simulink model "ClosedLoopPMSM_PID_asmo"  (R2023b)
settings: Solver=ode4  StartTime=0.0  StopTime=2.5  FixedStep=1e-6  RelTol=1e-4
InitFcn:
  | Vdc=24;
  | Rs=0.05734;
  | Ld=1.8166e-05;
  | Lq=1.8166e-05;
  | Ls=1.8166e-05;
  | pm=0.0185;
  | P=14;
  | B=1e-4;
  | J=2.94e-5;
  | Tpwm=30e-6;
  | 
  | fc=20;
  | mag_vel=100;
undefined symbols (not defined in the file): DiscIntNeverNeededParam
libraries: simulink x4, slpidlib x3, spsThreePhaseVIMeasurementLib x2, spsDCVoltageSourceLib x2, spsThreeLevelBridgeLib x1, spsUniversalBridgeLib x1, spsPermanentMagnetSynchronousMachineLib x1, sps_lib x1
settings Model: Creator=Admin  LastModifiedBy=Admin
settings SolverCC: AlgebraicLoopSolver=TrustRegion
settings DataIOCC: ReturnWorkspaceOutputs=off
settings OptimizationCC: LifeSpan=inf
settings DebuggingCC: UnconnectedInputMsg=warning  UnconnectedOutputMsg=warning  UnconnectedLineMsg=warning  SFUnexpectedBacktrackingDiag=warning  SFNoUnconditionalDefaultTransitionDiag=warning  ArithmeticOperatorsInVariantConditions=warning
settings ModelReferenceCC: EnableRefExpFcnMdlSchedulingChecks=on
settings SFSimCC: SimUseLocalCustomCode=off  CustomCodeUndefinedFunction=UseInterfaceOnly
settings RTWCC: RTWUseLocalCustomCode=off
settings CodeAppCC: StateflowObjectComments=on
settings GRTTargetCC: TargetLangStandard=C89/C90 (ANSI)
settings ConfigComp: CovMetricSettings=dw  CovSaveCumulativeToWorkspaceVar=on  CovSaveSingleToWorkspaceVar=on  CovExternalEMLEnable=off
settings SimscapeCC: SimscapeNormalizeSystem=off

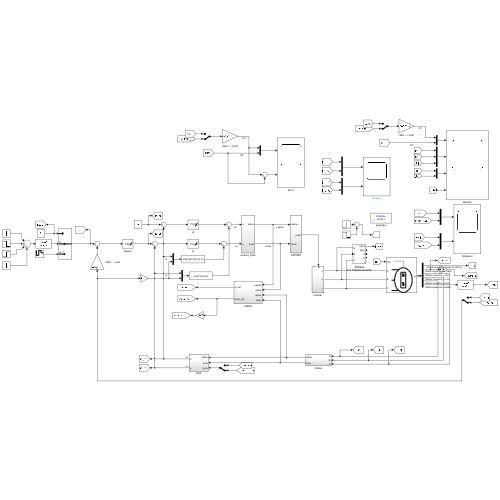
[thumbnail: Simulink's stored preview of the top-level diagram]
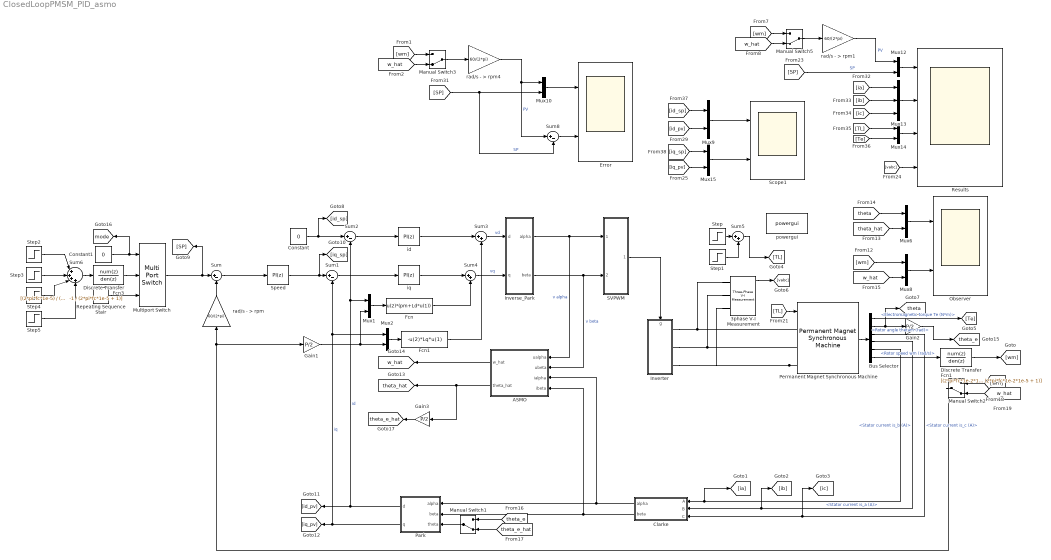
== system ClosedLoopPMSM_PID_asmo ==
  3phase V-I Measurement : spsThreePhaseVIMeasurementLib/Three-Phase V-I Measurement  VoltageMeasurement=phase-to-phase  SetLabelV=off  LabelV=Vabc  Vpu=off  VpuLL=off  CurrentMeasurement=yes  SetLabelI=off  LabelI=Iabc  Ipu=off  Pbase=100e6  Vbase=500e3  OutputType=Complex  PhasorSimulation=off  PSBequivalent=0
  ASMO : Subsystem
  Bus Selector : BusSelector  OutputSignals=Electromagnetic torque Te (N*m),Rotor angle thetam (rad),Stator current is_c (A),Stator current is_b (A),Stator current is_a (A),Rotor speed wm (rad/s)
  Clarke : Subsystem
  Constant : Constant  Value=0
  Constant1 : Constant  Value=0
  Discrete Transfer Fcn1 : DiscreteTransferFcn  Numerator=[(2*pi*fc*1e-2*1e-5) / (2*pi*fc*1e-2*1e-5 + 1)]  Denominator="[1   -1 / (2*pi*fc*1e-2*1e-5 + 1)]"
  Discrete Transfer Fcn3 : DiscreteTransferFcn  Numerator=[(2*pi*fc*1e-5) / (2*pi*fc*1e-5 + 1)]  Denominator="[1   -1 / (2*pi*fc*1e-5 + 1)]"
  Error : Scope  NumInputPorts=2
  Fcn : Fcn  Expr=u(2)*(pm+Ld*u(1))
  Fcn1 : Fcn  Expr=-u(2)*Lq*u(1)
  Gain1 : Gain  Gain=P/2
  Gain2 : Gain  Gain=P/2
  Gain3 : Gain  Gain=P/2
  Inverse_Park : Subsystem
  Inverter : Subsystem
      settings: PortSchema="{\"entries\":[{\"content\":{\"sides\":[{\"content\":{},\"type\":\"ConnectorPlacement.EquallySpacedRectSide\",\"uuid\":\"187c6bc1-a8de-4289-8015-4317398378bc\"},{\"content\":{\"connectorIds\":[\"RConn1\",\"RConn2\",\"RConn3\"],\"side\":\"RIGHT\"},\"type\":\"ConnectorPlacement.EquallySpacedRectSide\",\"uuid\":\"9f177a2c-a1b4-485f-9b91-a35efcc62074\"},{\"content\":{\"connectorIds\":[\"In1\"],\"side\":\"TOP\"},\"type\":\"ConnectorPlacement.EquallySpacedRectSide\",\"uuid\":\"7cd38b0a-0afe-4879-8b43-8c0c1c17e55c\"}]},\"type\":\"ConnectorPlacement.EquallySpacedConnector\",\"uuid\":\"53672e9b-5b63-4df3-a21b-cd886d268e09\"}],\"packageUris\":[\"http://schema.mathworks.com/mf0/Connector/R2020b\"],\"version\":\"1.0\"}"
  Manual Switch{1..3,5} (4 alike) : ManualSwitch  CurrentSetting=0
  Multiport Switch : MultiPortSwitch  DataPortOrder=Zero-based contiguous  Inputs=2  zeroidx=on  SaturateOnIntegerOverflow=off  InputSameDT=off
  Mux{1..2,6,8..10,12,14..15} (9 alike) : Mux  Inputs=2
  Mux13 : Mux  Inputs=3
  Observer : Scope  NumInputPorts=2
  Park : Subsystem
  Permanent Magnet Synchronous Machine : spsPermanentMagnetSynchronousMachineLib/Permanent Magnet Synchronous Machine  NbPhases=3  FluxDistribution=Sinusoidal  RotorType=Salient-pole  MechanicalLoad=Torque Tm  PresetModel=No  ShowDetailedParameters=on  MeasurementBus=off  Resistance=Rs  Inductance=8.5e-3  dqInductances=[Ld,Lq]  La=0.000395  MachineConstant=Flux linkage established by magnets (V.s)  Flux=pm  VoltageCst=23.4887  TorqueCst=0.19425  Flat=120  Mechanical=[J B P/2]  PolePairs=4  InitialConditions=[0,0, 0,0]  InitialConditions5ph=[0 0 0 0 0 0]  RefAngle=Aligned with phase A axis (original Park)  IterativeDiscreteModel=Trapezoidal non iterative  TsBlock=-1  TsPowergui=0
  Repeating Sequence Stair : simulink/Sources/Repeating Sequence Stair  OutValues=[50 150 100].'  tsamp=1  OutMin=[]  OutMax=[]  OutDataTypeStr=double  OutputDataTypeScalingMode=double  OutDataType=fixdt(0,8)  ConRadixGroup=Best Precision: Vector-wise  OutScaling=2^-12
  Results : Scope  NumInputPorts=4
  SVPWM : Subsystem
  Scope1 : Scope  NumInputPorts=2
  Speed : slpidlib/PID Controller  Controller=PI  Form=Parallel  TimeDomain=Discrete-time  UseExternalTs=off  SampleTime=-1  IntegratorMethod=Forward Euler  FilterMethod=Forward Euler  ControllerParametersSource=internal  P=3e-1  I=150e-1  UseKiTs=off  D=1e0  N=1  UseFilter=on  TunerSelectOption=Transfer Function Based (PID Tuner App)  ZeroCross=off  InitialConditionSource=internal  InitialConditionForIntegrator=0  InitialConditionForFilter=0  DifferentiatorICPrevScaledInput=0  ExternalReset=none  TrackingMode=off  Kt=1  LimitOutput=on  SatLimitsSource=internal  UpperSaturationLimit=10  LowerSaturationLimit=-10  LinearizeAsGain=off  AntiWindupMode=clamping  Kb=1  LimitIntegrator=off  UpperIntegratorSaturationLimit=10  LowerIntegratorSaturationLimit=-10  POutMin=[]  POutMax=[]  IOutMin=[]  IOutMax=[]  DOutMin=[]  DOutMax=[]  NOutMin=[]  NOutMax=[]  SumOutMin=[]  SumOutMax=[]  SaturationOutMin=[]  SaturationOutMax=[]  PParamMin=[]  PParamMax=[]  IParamMin=[]  IParamMax=[]  DParamMin=[]  DParamMax=[]  NParamMin=[]  NParamMax=[]  KbParamMin=[]  KbParamMax=[]  KtParamMin=[]  KtParamMax=[]  KbOutMin=[]  KbOutMax=[]  KtOutMin=[]  KtOutMax=[]  IntegratorOutMin=[]  IntegratorOutMax=[]  FilterOutMin=[]  FilterOutMax=[]  SumI1OutMin=[]  SumI1OutMax=[]  SumI2OutMin=[]  SumI2OutMax=[]  SumI3OutMin=[]  SumI3OutMax=[]  SumI4OutMin=[]  SumI4OutMax=[]  SumDOutMin=[]  SumDOutMax=[]  DifferentiatorOutMin=[]  DifferentiatorOutMax=[]  FilterDiffOutCoefMin=[]  FilterDiffOutCoefMax=[]  ReciprocalOutMin=[]  ReciprocalOutMax=[]  SumDenOutMin=[]  SumDenOutMax=[]  SumNumOutMin=[]  SumNumOutMax=[]  DivideOutMin=[]  DivideOutMax=[]  UdiffTsProdOutMin=[]  UdiffTsProdOutMax=[]  NTsProdOutMin=[]  NTsProdOutMax=[]  UintegralTsProdOutMin=[]  UintegralTsProdOutMax=[]  UngainTsProdOutMin=[]  UngainTsProdOutMax=[]  ClampingZeroOutDataTypeStr=Inherit: Inherit via back propagation  ClampingZeroOutMin=[]  ClampingZeroOutMax=[]  FilterDenConstantOutDataTypeStr=Inherit: Inherit via back propagation  FilterDenConstantOutMin=[]  FilterDenConstantOutMax=[]  PCopyOutDataTypeStr=Inherit: Inherit via back propagation  PCopyOutMin=[]  PCopyOutMax=[]  NCopyOutDataTypeStr=Inherit: Inherit via back propagation  NCopyOutMin=[]  NCopyOutMax=[]  IntegratorContinuousStateAttributes=''  IntegratorStateMustResolveToSignalObject=off  IntegratorRTWStateStorageClass=Auto  FilterContinuousStateAttributes=''  FilterStateMustResolveToSignalObject=off  FilterRTWStateStorageClass=Auto  ParallelPVariant=InternalParameters  IdealPVariant=Disabled  IVariant=InternalParameters  DVariant=Disabled  IntegratorVariant=Discrete  SatVariant=Enabled  AWVariant=DiscClampingParallel  PCopyVariant=Disabled  TRVariant=Disabled  FdbkBlocksVariant=Forward  IdealPFdbkVariant=Disabled  SatFdbkVariant=Disabled  DerivativeFilterVariant=Disabled  NVariant=Disabled  NCopyVariant=Disabled_SignalSpec  FilterICVariant=Disabled  IntegratorICVariant=InternalICs  ExternalResetVariant=Disabled  TRSumVariant=Passthrough  SumFdbkVariant=Disabled  SumVariant=Sum_PI  TsampFilterVariant=InternalTs  TsampNgainVariant=Passthrough  TsampIntegralVariant=Disabled_SignalSpec  ExternalSaturationOutDataTypeStr=Inherit: Same as second input
  Step : Step  Time=0.1  After=0.1  SampleTime=0
  Step1 : Step  Time=0.15  After=-0.1  SampleTime=0
  Step2 : Step  Time=0.1  After=mag_vel*3  SampleTime=0
  Step3 : Step  Time=1.0  After=-200  SampleTime=0
  Step4 : Step  Time=1.5  After=+100  SampleTime=0
  Step5 : Step  Time=2  After=-200  SampleTime=0
  Sum{,1..2,8} (4 alike) : Sum  Inputs=|+-
  Sum3 : Sum  Inputs=|++
  Sum4 : Sum  Inputs=|++
  Sum5 : Sum  Inputs=|++
  Sum6 : Sum  Inputs=|++++
  id : slpidlib/PID Controller  Controller=PI  Form=Parallel  TimeDomain=Discrete-time  UseExternalTs=off  SampleTime=-1  IntegratorMethod=Forward Euler  FilterMethod=Forward Euler  ControllerParametersSource=internal  P=0.02283e5  I=72.06e3  UseKiTs=off  D=0  N=100  UseFilter=on  TunerSelectOption=Transfer Function Based (PID Tuner App)  ZeroCross=off  InitialConditionSource=internal  InitialConditionForIntegrator=0  InitialConditionForFilter=0  DifferentiatorICPrevScaledInput=0  ExternalReset=none  TrackingMode=off  Kt=1  LimitOutput=on  SatLimitsSource=internal  UpperSaturationLimit=8  LowerSaturationLimit=-8  LinearizeAsGain=off  AntiWindupMode=clamping  Kb=1  LimitIntegrator=on  UpperIntegratorSaturationLimit=10  LowerIntegratorSaturationLimit=-10  POutMin=[]  POutMax=[]  IOutMin=[]  IOutMax=[]  DOutMin=[]  DOutMax=[]  NOutMin=[]  NOutMax=[]  SumOutMin=[]  SumOutMax=[]  SaturationOutMin=[]  SaturationOutMax=[]  PParamMin=[]  PParamMax=[]  IParamMin=[]  IParamMax=[]  DParamMin=[]  DParamMax=[]  NParamMin=[]  NParamMax=[]  KbParamMin=[]  KbParamMax=[]  KtParamMin=[]  KtParamMax=[]  KbOutMin=[]  KbOutMax=[]  KtOutMin=[]  KtOutMax=[]  IntegratorOutMin=[]  IntegratorOutMax=[]  FilterOutMin=[]  FilterOutMax=[]  SumI1OutMin=[]  SumI1OutMax=[]  SumI2OutMin=[]  SumI2OutMax=[]  SumI3OutMin=[]  SumI3OutMax=[]  SumI4OutMin=[]  SumI4OutMax=[]  SumDOutMin=[]  SumDOutMax=[]  DifferentiatorOutMin=[]  DifferentiatorOutMax=[]  FilterDiffOutCoefMin=[]  FilterDiffOutCoefMax=[]  ReciprocalOutMin=[]  ReciprocalOutMax=[]  SumDenOutMin=[]  SumDenOutMax=[]  SumNumOutMin=[]  SumNumOutMax=[]  DivideOutMin=[]  DivideOutMax=[]  UdiffTsProdOutMin=[]  UdiffTsProdOutMax=[]  NTsProdOutMin=[]  NTsProdOutMax=[]  UintegralTsProdOutMin=[]  UintegralTsProdOutMax=[]  UngainTsProdOutMin=[]  UngainTsProdOutMax=[]  ClampingZeroOutDataTypeStr=Inherit: Inherit via back propagation  ClampingZeroOutMin=[]  ClampingZeroOutMax=[]  FilterDenConstantOutDataTypeStr=Inherit: Inherit via back propagation  FilterDenConstantOutMin=[]  FilterDenConstantOutMax=[]  PCopyOutDataTypeStr=Inherit: Inherit via back propagation  PCopyOutMin=[]  PCopyOutMax=[]  NCopyOutDataTypeStr=Inherit: Inherit via back propagation  NCopyOutMin=[]  NCopyOutMax=[]  IntegratorContinuousStateAttributes=''  IntegratorStateMustResolveToSignalObject=off  IntegratorRTWStateStorageClass=Auto  FilterContinuousStateAttributes=''  FilterStateMustResolveToSignalObject=off  FilterRTWStateStorageClass=Auto  ParallelPVariant=InternalParameters  IdealPVariant=Disabled  IVariant=InternalParameters  DVariant=Disabled  IntegratorVariant=Discrete  SatVariant=Enabled  AWVariant=DiscClampingParallel  PCopyVariant=Disabled  TRVariant=Disabled  FdbkBlocksVariant=Forward  IdealPFdbkVariant=Disabled  SatFdbkVariant=Disabled  DerivativeFilterVariant=Disabled  NVariant=Disabled  NCopyVariant=Disabled_SignalSpec  FilterICVariant=Disabled  IntegratorICVariant=InternalICs  ExternalResetVariant=Disabled  TRSumVariant=Passthrough  SumFdbkVariant=Disabled  SumVariant=Sum_PI  TsampFilterVariant=InternalTs  TsampNgainVariant=Passthrough  TsampIntegralVariant=Disabled_SignalSpec  ExternalSaturationOutDataTypeStr=Inherit: Same as second input
  iq : slpidlib/PID Controller  Controller=PI  Form=Parallel  TimeDomain=Discrete-time  UseExternalTs=off  SampleTime=-1  IntegratorMethod=Forward Euler  FilterMethod=Forward Euler  ControllerParametersSource=internal  P=0.02283e5  I=72.06e3  UseKiTs=off  D=0  N=100  UseFilter=on  TunerSelectOption=Transfer Function Based (PID Tuner App)  ZeroCross=off  InitialConditionSource=internal  InitialConditionForIntegrator=0  InitialConditionForFilter=0  DifferentiatorICPrevScaledInput=0  ExternalReset=none  TrackingMode=off  Kt=1  LimitOutput=on  SatLimitsSource=internal  UpperSaturationLimit=8  LowerSaturationLimit=-8  LinearizeAsGain=off  AntiWindupMode=clamping  Kb=1  LimitIntegrator=on  UpperIntegratorSaturationLimit=10  LowerIntegratorSaturationLimit=-10  POutMin=[]  POutMax=[]  IOutMin=[]  IOutMax=[]  DOutMin=[]  DOutMax=[]  NOutMin=[]  NOutMax=[]  SumOutMin=[]  SumOutMax=[]  SaturationOutMin=[]  SaturationOutMax=[]  PParamMin=[]  PParamMax=[]  IParamMin=[]  IParamMax=[]  DParamMin=[]  DParamMax=[]  NParamMin=[]  NParamMax=[]  KbParamMin=[]  KbParamMax=[]  KtParamMin=[]  KtParamMax=[]  KbOutMin=[]  KbOutMax=[]  KtOutMin=[]  KtOutMax=[]  IntegratorOutMin=[]  IntegratorOutMax=[]  FilterOutMin=[]  FilterOutMax=[]  SumI1OutMin=[]  SumI1OutMax=[]  SumI2OutMin=[]  SumI2OutMax=[]  SumI3OutMin=[]  SumI3OutMax=[]  SumI4OutMin=[]  SumI4OutMax=[]  SumDOutMin=[]  SumDOutMax=[]  DifferentiatorOutMin=[]  DifferentiatorOutMax=[]  FilterDiffOutCoefMin=[]  FilterDiffOutCoefMax=[]  ReciprocalOutMin=[]  ReciprocalOutMax=[]  SumDenOutMin=[]  SumDenOutMax=[]  SumNumOutMin=[]  SumNumOutMax=[]  DivideOutMin=[]  DivideOutMax=[]  UdiffTsProdOutMin=[]  UdiffTsProdOutMax=[]  NTsProdOutMin=[]  NTsProdOutMax=[]  UintegralTsProdOutMin=[]  UintegralTsProdOutMax=[]  UngainTsProdOutMin=[]  UngainTsProdOutMax=[]  ClampingZeroOutDataTypeStr=Inherit: Inherit via back propagation  ClampingZeroOutMin=[]  ClampingZeroOutMax=[]  FilterDenConstantOutDataTypeStr=Inherit: Inherit via back propagation  FilterDenConstantOutMin=[]  FilterDenConstantOutMax=[]  PCopyOutDataTypeStr=Inherit: Inherit via back propagation  PCopyOutMin=[]  PCopyOutMax=[]  NCopyOutDataTypeStr=Inherit: Inherit via back propagation  NCopyOutMin=[]  NCopyOutMax=[]  IntegratorContinuousStateAttributes=''  IntegratorStateMustResolveToSignalObject=off  IntegratorRTWStateStorageClass=Auto  FilterContinuousStateAttributes=''  FilterStateMustResolveToSignalObject=off  FilterRTWStateStorageClass=Auto  ParallelPVariant=InternalParameters  IdealPVariant=Disabled  IVariant=InternalParameters  DVariant=Disabled  IntegratorVariant=Discrete  SatVariant=Enabled  AWVariant=DiscClampingParallel  PCopyVariant=Disabled  TRVariant=Disabled  FdbkBlocksVariant=Forward  IdealPFdbkVariant=Disabled  SatFdbkVariant=Disabled  DerivativeFilterVariant=Disabled  NVariant=Disabled  NCopyVariant=Disabled_SignalSpec  FilterICVariant=Disabled  IntegratorICVariant=InternalICs  ExternalResetVariant=Disabled  TRSumVariant=Passthrough  SumFdbkVariant=Disabled  SumVariant=Sum_PI  TsampFilterVariant=InternalTs  TsampNgainVariant=Passthrough  TsampIntegralVariant=Disabled_SignalSpec  ExternalSaturationOutDataTypeStr=Inherit: Same as second input
  powergui : sps_lib/powergui  Priority=1  SimulationMode=Discrete  SampleTime=1e-6  frequency=60  Iterations=50  frequencyindice=0  Pbase=100e6  ErrMax=1e-4  UnitsV=kV  UnitsW=MW  buscounter=0  FunctionMessages=off  echomessages=off  EnableUseOfTLC=off  CurrentSourceSwitches=on  DisableSnubberDevices=off  DisableRonSwitches=off  DisableVfSwitches=off  DisplayEquations=off  AutomaticDiscreteSolvers=off  SolverType=Tustin/Backward Euler (TBE)  Interpol=off  ExternalGateDelay=off  methode=off  Ts=100  x0status=blocks  SPID=on  SwTol=0  HookPort=off  NonlinearTolerance=1e-4  nMaxIteration=100  ContinueOnMaxIteration=off  RestoreLinks=warning  ResistiveCurrentMeasurement=off  Frange=[0:2:500]  Ylog=off  Xlog=on  ShowGrid=off  save=off  variable=ZData  structure=0  ZoomFFT=off  StartTime=0.0  cycles=1  DisplayStyle=1  fundamental=60  FreqAxis=off  MaxFrequency=1000  frequencyindicesteady=1  RmsSteady=1  display=off
  rad/s - > rpm : Gain  Gain=60/(2*pi)
  rad/s - > rpm1 : Gain  Gain=60/(2*pi)
  rad/s - > rpm4 : Gain  Gain=60/(2*pi)
  tag scope: mode=global, theta=global, theta_e=global, theta_e_hat=global, theta_hat=global, w_hat=global
  wires:
  Constant/1 -> Sum2/1, [id_sp]
  Park/1(d) -> Sum2/2, Mux1/1, [id_pv]  "id"
  Park/2(q) -> Sum1/2, Mux2/1, [iq_pv]  "iq"
  Mux1/1 -> Fcn/1
  Mux2/1 -> Fcn1/1
  Permanent Magnet Synchronous Machine/1 -> Bus Selector/1
  Bus Selector/3 -> Clarke/3(C), [ic]  "<Stator current is_c (A)>"
  Bus Selector/4 -> Clarke/2(B), [ib]  "<Stator current is_b (A)>"
  Bus Selector/5 -> Clarke/1(A), [ia]  "<Stator current is_a (A)>"
  rad/s - > rpm/1 -> Sum/2
  Gain1/1 -> Mux1/2, Mux2/2
  Sum5/1 -> [TL]
  Bus Selector/1 -> [Te]  "<Electromagnetic torque Te (N*m)>"
  3phase V-I Measurement/1 -> [vabc]
  Sum3/1 -> Inverse_Park/1(d)  "vd"
  Sum4/1 -> Inverse_Park/2(q)  "vq"
  SVPWM/1(pulse) -> Inverter/1(g)
  Inverse_Park/1(alpha) -> ASMO/1(ualpha), SVPWM/1(valpha)  "v alpha"
  Inverse_Park/2(beta) -> ASMO/2(ubeta), SVPWM/2(vbeta)  "v beta"
  Step1/1 -> Sum5/2
  Step/1 -> Sum5/1
  Gain2/1 -> [theta_e]
  Discrete Transfer Fcn3/1 -> Multiport Switch/2
  Constant1/1 -> [mode], Multiport Switch/1
  Multiport Switch/1 -> Sum/1, [SP]
  Step3/1 -> Sum6/2
  Step2/1 -> Sum6/1
  Sum6/1 -> Discrete Transfer Fcn3/1
  [theta_e_hat] -> Manual Switch1/2
  [theta_e] -> Manual Switch1/1
  Manual Switch2/1 -> Gain1/1, rad/s - > rpm/1
  Bus Selector/6 -> Discrete Transfer Fcn1/1  "<Rotor speed wm (rad/s)>"
  [wm] -> Manual Switch2/1
  [w_hat] -> Manual Switch2/2
  Sum2/1 -> id/1
  Sum1/1 -> iq/1
  Fcn/1 -> Sum4/2
  Fcn1/1 -> Sum3/2
  Gain3/1 -> [theta_e_hat]
  ASMO/2(theta_hat) -> [theta_hat], Gain3/1
  Manual Switch1/1 -> Park/3(theta)
  Clarke/2(beta) -> ASMO/4(ibeta), Park/2(beta)
  Clarke/1(alpha) -> ASMO/3(ialpha), Park/1(alpha)
  Repeating Sequence Stair/1 -> Multiport Switch/3
  Sum/1 -> Speed/1
  ASMO/1(w_hat) -> [w_hat]
  id/1 -> Sum3/1
  iq/1 -> Sum4/1
  Speed/1 -> [iq_sp], Sum1/1
  Discrete Transfer Fcn1/1 -> [wm]
  Bus Selector/2 -> [theta], Gain2/1  "<Rotor angle thetam (rad)>"
  [TL] -> Permanent Magnet Synchronous Machine/1
  [iq_pv] -> Mux15/2
  rad/s - > rpm1/1 -> Mux12/1  "PV"
  Mux9/1 -> Scope1/1
  Mux12/1 -> Results/1
  [ib] -> Mux13/2
  [ia] -> Mux13/1
  [id_pv] -> Mux9/2
  Mux14/1 -> Results/3
  Mux13/1 -> Results/2
  [ic] -> Mux13/3
  Mux15/1 -> Scope1/2
  [id_sp] -> Mux9/1
  [Te] -> Mux14/2
  [SP] -> Mux12/2  "SP"
  Sum8/1 -> Error/2
  [SP] -> Sum8/2, Mux10/2  "SP"
  [iq_sp] -> Mux15/1
  Mux10/1 -> Error/1
  Manual Switch3/1 -> rad/s - > rpm4/1
  rad/s - > rpm4/1 -> Sum8/1, Mux10/1  "PV"
  [TL] -> Mux14/1
  [vabc] -> Results/4
  [w_hat] -> Manual Switch5/2
  [wm] -> Manual Switch5/1
  Manual Switch5/1 -> rad/s - > rpm1/1
  [w_hat] -> Manual Switch3/2
  [wm] -> Manual Switch3/1
  [theta] -> Mux6/1
  [w_hat] -> Mux8/2
  [wm] -> Mux8/1
  Mux6/1 -> Observer/1
  [theta_hat] -> Mux6/2
  Mux8/1 -> Observer/2
  Step4/1 -> Sum6/3
  Step5/1 -> Sum6/4
  connections:
  3phase V-I Measurement/LConn1 -- Inverter/RConn1 -- Permanent Magnet Synchronous Machine/LConn1
  3phase V-I Measurement/LConn2 -- Inverter/RConn2 -- Permanent Magnet Synchronous Machine/LConn2
  Permanent Magnet Synchronous Machine/LConn3 -- Inverter/RConn3 -- 3phase V-I Measurement/LConn3

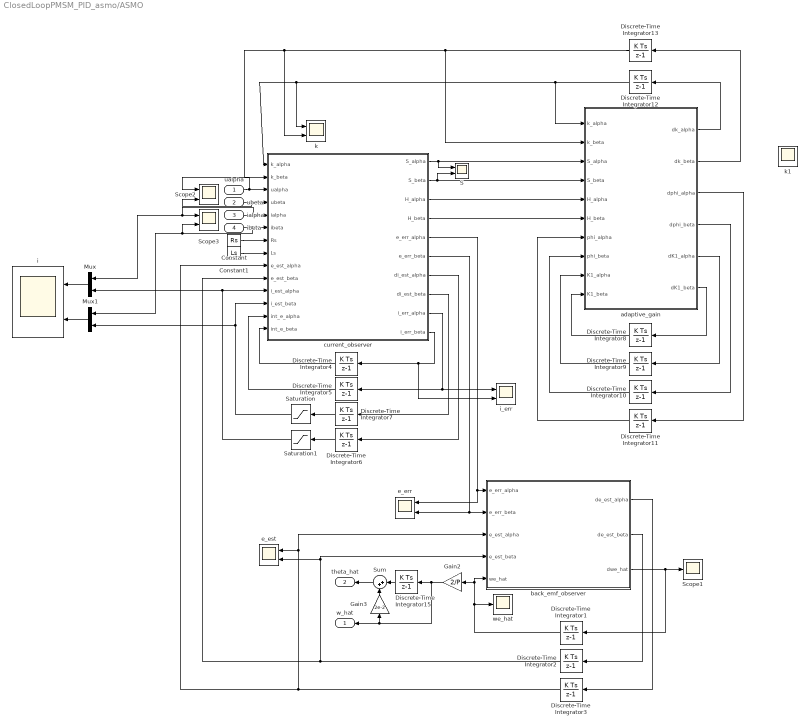
== system ClosedLoopPMSM_PID_asmo/ASMO ==
  ualpha : Inport
  ubeta : Inport  Port=2
  ialpha : Inport  Port=3
  ibeta : Inport  Port=4
  Constant : Constant  Value=Rs
  Constant1 : Constant  Value=Ls
  Discrete-Time Integrator1 : DiscreteIntegrator  gainval=2.5e2*3  SampleTime=-1  ICPrevOutput=DiscIntNeverNeededParam  ICPrevScaledInput=DiscIntNeverNeededParam
  Discrete-Time Integrator{2..5,8..11} (8 alike) : DiscreteIntegrator  SampleTime=-1  ICPrevOutput=DiscIntNeverNeededParam  ICPrevScaledInput=DiscIntNeverNeededParam
  Discrete-Time Integrator12 : DiscreteIntegrator  InitialCondition=50  SampleTime=-1  ICPrevOutput=DiscIntNeverNeededParam  ICPrevScaledInput=DiscIntNeverNeededParam
  Discrete-Time Integrator13 : DiscreteIntegrator  InitialCondition=50  SampleTime=-1  ICPrevOutput=DiscIntNeverNeededParam  ICPrevScaledInput=DiscIntNeverNeededParam
  Discrete-Time Integrator15 : DiscreteIntegrator  gainval=1  SampleTime=-1  ICPrevOutput=DiscIntNeverNeededParam  ICPrevScaledInput=DiscIntNeverNeededParam
  Discrete-Time Integrator6 : DiscreteIntegrator  gainval=1.0e-2*5  SampleTime=-1  ICPrevOutput=DiscIntNeverNeededParam  ICPrevScaledInput=DiscIntNeverNeededParam
  Discrete-Time Integrator7 : DiscreteIntegrator  gainval=1.0e-2*5  SampleTime=-1  ICPrevOutput=DiscIntNeverNeededParam  ICPrevScaledInput=DiscIntNeverNeededParam
  Gain2 : Gain  Gain=2/P
  Gain3 : Gain  Gain=2e-2
  Mux : Mux  Inputs=2
  Mux1 : Mux  Inputs=2
  S : Scope  NumInputPorts=2
  Saturation : Saturate  UpperLimit=1  LowerLimit=-1
  Saturation1 : Saturate  UpperLimit=1  LowerLimit=-1
  Scope1 : Scope
  Scope2 : Scope  NumInputPorts=2
  Scope3 : Scope  NumInputPorts=2
  Sum : Sum  Inputs=|++
  adaptive_gain : MATLAB Function  TreatAsAtomicUnit=on
  back_emf_observer : MATLAB Function  TreatAsAtomicUnit=on
  current_observer : MATLAB Function  TreatAsAtomicUnit=on
  e_err : Scope  NumInputPorts=2
  e_est : Scope  NumInputPorts=2
  i : Scope  NumInputPorts=2
  i_err : Scope  NumInputPorts=2
  k : Scope  NumInputPorts=2
  k1 : Scope  NumInputPorts=2
  we_hat : Scope
  w_hat : Outport
  theta_hat : Outport  Port=2
  wires:
  ualpha/1 -> Scope2/1, current_observer/3(ualpha)
  ubeta/1 -> current_observer/4(ubeta), Scope2/2
  ialpha/1 -> Scope3/1, Mux/1, current_observer/5(ialpha)
  ibeta/1 -> Scope3/2, Mux1/1, current_observer/6(ibeta)
  Constant/1 -> current_observer/7(Rs)
  Constant1/1 -> current_observer/8(Ls)
  current_observer/7(di_est_alpha) -> Discrete-Time Integrator6/1
  current_observer/8(di_est_beta) -> Discrete-Time Integrator7/1
  current_observer/1(S_alpha) -> adaptive_gain/3(S_alpha), S/1
  current_observer/2(S_beta) -> S/2, adaptive_gain/4(S_beta)
  current_observer/3(H_alpha) -> adaptive_gain/5(H_alpha)
  current_observer/4(H_beta) -> adaptive_gain/6(H_beta)
  adaptive_gain/3(dphi_alpha) -> Discrete-Time Integrator11/1
  adaptive_gain/4(dphi_beta) -> Discrete-Time Integrator10/1
  adaptive_gain/5(dK1_alpha) -> Discrete-Time Integrator9/1
  adaptive_gain/6(dK1_beta) -> Discrete-Time Integrator8/1
  adaptive_gain/1(dk_alpha) -> Discrete-Time Integrator12/1
  adaptive_gain/2(dk_beta) -> Discrete-Time Integrator13/1
  back_emf_observer/1(de_est_alpha) -> Discrete-Time Integrator3/1
  back_emf_observer/2(de_est_beta) -> Discrete-Time Integrator2/1
  Discrete-Time Integrator4/1 -> current_observer/14(int_e_beta)
  Discrete-Time Integrator5/1 -> current_observer/13(int_e_alpha)
  Discrete-Time Integrator7/1 -> Saturation/1
  Discrete-Time Integrator6/1 -> Saturation1/1
  Discrete-Time Integrator8/1 -> adaptive_gain/10(K1_beta)
  Discrete-Time Integrator9/1 -> adaptive_gain/9(K1_alpha)
  Discrete-Time Integrator10/1 -> adaptive_gain/8(phi_beta)
  Discrete-Time Integrator11/1 -> adaptive_gain/7(phi_alpha)
  Discrete-Time Integrator13/1 -> adaptive_gain/2(k_beta), k/2, current_observer/2(k_beta)
  Discrete-Time Integrator12/1 -> adaptive_gain/1(k_alpha), k/1, current_observer/1(k_alpha)
  current_observer/9(i_err_alpha) -> Discrete-Time Integrator5/1, i_err/1
  current_observer/10(i_err_beta) -> Discrete-Time Integrator4/1, i_err/2
  current_observer/5(e_err_alpha) -> e_err/1, back_emf_observer/1(e_err_alpha)
  current_observer/6(e_err_beta) -> e_err/2, back_emf_observer/2(e_err_beta)
  back_emf_observer/3(dwe_hat) -> Discrete-Time Integrator1/1, Scope1/1
  Discrete-Time Integrator2/1 -> current_observer/10(e_est_beta), e_est/2, back_emf_observer/4(e_est_beta)
  Discrete-Time Integrator3/1 -> current_observer/9(e_est_alpha), e_est/1, back_emf_observer/3(e_est_alpha)
  Discrete-Time Integrator15/1 -> Sum/1
  Sum/1 -> theta_hat/1
  Gain2/1 -> Gain3/1, w_hat/1, Discrete-Time Integrator15/1
  Gain3/1 -> Sum/2
  Mux/1 -> i/1
  Mux1/1 -> i/2
  Discrete-Time Integrator1/1 -> we_hat/1, back_emf_observer/5(we_hat), Gain2/1
  Saturation/1 -> current_observer/12(i_est_beta), Mux1/2
  Saturation1/1 -> current_observer/11(i_est_alpha), Mux/2

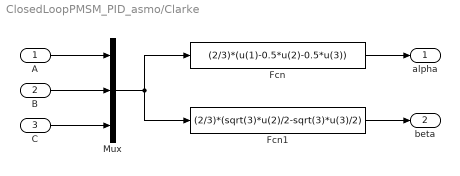
== system ClosedLoopPMSM_PID_asmo/Clarke ==
  A : Inport
  B : Inport  Port=2
  C : Inport  Port=3
  Fcn : Fcn  Expr=(2/3)*(u(1)-0.5*u(2)-0.5*u(3))
  Fcn1 : Fcn  Expr=(2/3)*(sqrt(3)*u(2)/2-sqrt(3)*u(3)/2)
  Mux : Mux  Inputs=3
  alpha : Outport
  beta : Outport  Port=2
  wires:
  B/1 -> Mux/2
  A/1 -> Mux/1
  C/1 -> Mux/3
  Mux/1 -> Fcn1/1, Fcn/1
  Fcn/1 -> alpha/1
  Fcn1/1 -> beta/1

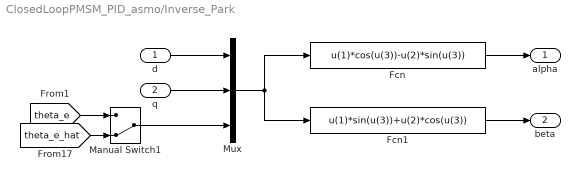
== system ClosedLoopPMSM_PID_asmo/Inverse_Park ==
  d : Inport
  q : Inport  Port=2
  Fcn : Fcn  Expr=u(1)*cos(u(3))-u(2)*sin(u(3))
  Fcn1 : Fcn  Expr=u(1)*sin(u(3))+u(2)*cos(u(3))
  Manual Switch1 : ManualSwitch  CurrentSetting=0
  Mux : Mux  Inputs=3
  alpha : Outport
  beta : Outport  Port=2
  wires:
  Fcn1/1 -> beta/1
  d/1 -> Mux/1
  q/1 -> Mux/2
  Mux/1 -> Fcn1/1, Fcn/1
  Fcn/1 -> alpha/1
  [theta_e] -> Manual Switch1/1
  [theta_e_hat] -> Manual Switch1/2
  Manual Switch1/1 -> Mux/3

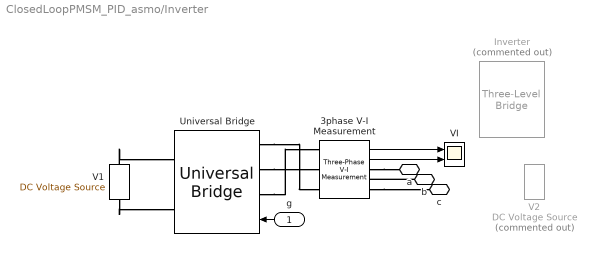
== system ClosedLoopPMSM_PID_asmo/Inverter ==
  g : Inport
  3phase V-I Measurement : spsThreePhaseVIMeasurementLib/Three-Phase V-I Measurement  VoltageMeasurement=phase-to-phase  SetLabelV=off  LabelV=Vabc  Vpu=off  VpuLL=off  CurrentMeasurement=yes  SetLabelI=off  LabelI=Iabc  Ipu=off  Pbase=100e6  Vbase=500e3  OutputType=Complex  PhasorSimulation=off  PSBequivalent=0
  Inverter : spsThreeLevelBridgeLib/Three-Level Bridge  Commented=on  Arms=3  SnubberResistance=1e5  SbubberCapacitance=1e-8  Device=IGBT / Diodes  Ron=0.2e-7  ForwardVoltages=[0.1 0.1]  Measurements=All voltages and currents
      settings: AttributesFormatString=\n
  Universal Bridge : spsUniversalBridgeLib/Universal Bridge  Arms=3  SnubberResistance=1e5  SnubberCapacitance=1e-8  Device=MOSFET / Diodes  Ron=0.2e-7  Lon=0  ForwardVoltages="[  0  0  ]"  ForwardVoltage=0  GTOparameters=[ 10e-6 , 20e-6 ]  IGBTparameters=[ 1e-6 , 2e-6 ]  Measurements=All voltages and currents  Measurements_2=None  converterType=Rectifier
  V1 : spsDCVoltageSourceLib/DC Voltage Source  Amplitude=Vdc  Measurements=None
  V2 : spsDCVoltageSourceLib/DC Voltage Source  Commented=on  Amplitude=Vdc/2  Measurements=None
  VI : Scope  NumInputPorts=2
  a : PMIOPort  Side=Right
  b : PMIOPort  Port=2  Side=Right
  c : PMIOPort  Port=3  Side=Right
  wires:
  3phase V-I Measurement/2 -> VI/2
  3phase V-I Measurement/1 -> VI/1
  g/1 -> Universal Bridge/1
  connections:
  3phase V-I Measurement/RConn3 -- c/RConn1
  b/RConn1 -- 3phase V-I Measurement/RConn2
  3phase V-I Measurement/RConn1 -- a/RConn1
  Universal Bridge/LConn3 -- 3phase V-I Measurement/LConn3
  Universal Bridge/LConn2 -- 3phase V-I Measurement/LConn2
  Universal Bridge/LConn1 -- 3phase V-I Measurement/LConn1
  V1/RConn1 -- Universal Bridge/RConn1
  V1/LConn1 -- Universal Bridge/RConn2

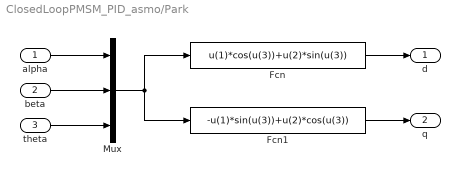
== system ClosedLoopPMSM_PID_asmo/Park ==
  alpha : Inport
  beta : Inport  Port=2
  theta : Inport  Port=3
  Fcn : Fcn  Expr=u(1)*cos(u(3))+u(2)*sin(u(3))
  Fcn1 : Fcn  Expr=-u(1)*sin(u(3))+u(2)*cos(u(3))
  Mux : Mux  Inputs=3
  d : Outport
  q : Outport  Port=2
  wires:
  beta/1 -> Mux/2
  alpha/1 -> Mux/1
  Mux/1 -> Fcn1/1, Fcn/1
  Fcn/1 -> d/1
  Fcn1/1 -> q/1
  theta/1 -> Mux/3

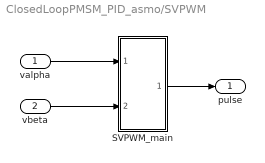
== system ClosedLoopPMSM_PID_asmo/SVPWM ==
  valpha : Inport
  vbeta : Inport  Port=2
  SVPWM_main : Subsystem
  pulse : Outport
  wires:
  SVPWM_main/1(pulse) -> pulse/1
  valpha/1 -> SVPWM_main/1(Ualpha)
  vbeta/1 -> SVPWM_main/2(Ubeta)

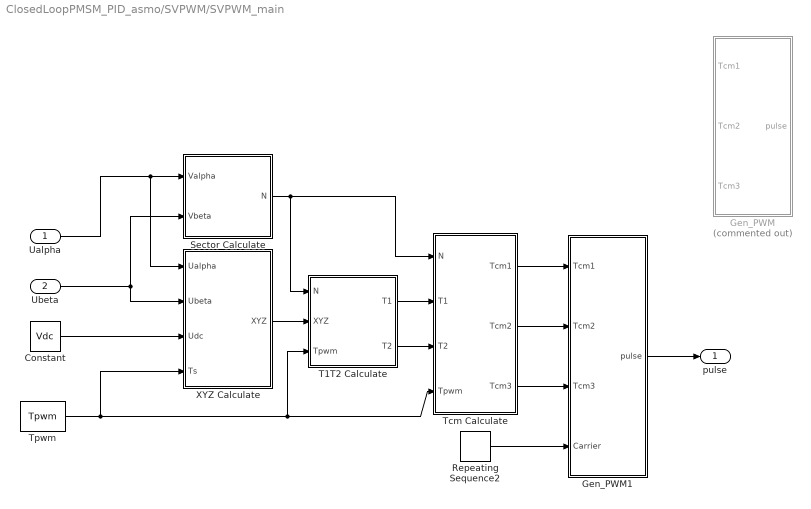
== system ClosedLoopPMSM_PID_asmo/SVPWM/SVPWM_main ==
  Ualpha : Inport
  Ubeta : Inport  Port=2
  Constant : Constant  Value=Vdc
  Gen_PWM : Subsystem  Commented=on
  Gen_PWM1 : Subsystem
  Repeating Sequence2 : simulink/Sources/Repeating Sequence  rep_seq_t=[0 Tpwm/2 Tpwm]  rep_seq_y=[0 Tpwm/8 0]
  Sector Calculate : MATLAB Function  TreatAsAtomicUnit=on
  T1T2 Calculate : MATLAB Function  TreatAsAtomicUnit=on
  Tcm Calculate : MATLAB Function  TreatAsAtomicUnit=on
  Tpwm : Constant  Value=Tpwm
  XYZ Calculate : MATLAB Function  TreatAsAtomicUnit=on
  pulse : Outport
  wires:
  Tpwm/1 -> XYZ Calculate/4(Ts), T1T2 Calculate/3(Tpwm), Tcm Calculate/4(Tpwm)
  Sector Calculate/1(N) -> Tcm Calculate/1(N), T1T2 Calculate/1(N)
  Ualpha/1 -> Sector Calculate/1(Valpha), XYZ Calculate/1(Ualpha)
  T1T2 Calculate/1(T1) -> Tcm Calculate/2(T1)
  Ubeta/1 -> Sector Calculate/2(Vbeta), XYZ Calculate/2(Ubeta)
  XYZ Calculate/1(XYZ) -> T1T2 Calculate/2(XYZ)
  Constant/1 -> XYZ Calculate/3(Udc)
  T1T2 Calculate/2(T2) -> Tcm Calculate/3(T2)
  Tcm Calculate/1(Tcm1) -> Gen_PWM1/1(Tcm1)
  Tcm Calculate/2(Tcm2) -> Gen_PWM1/2(Tcm2)
  Tcm Calculate/3(Tcm3) -> Gen_PWM1/3(Tcm3)
  Repeating Sequence2/1 -> Gen_PWM1/4(Carrier)
  Gen_PWM1/1(pulse) -> pulse/1

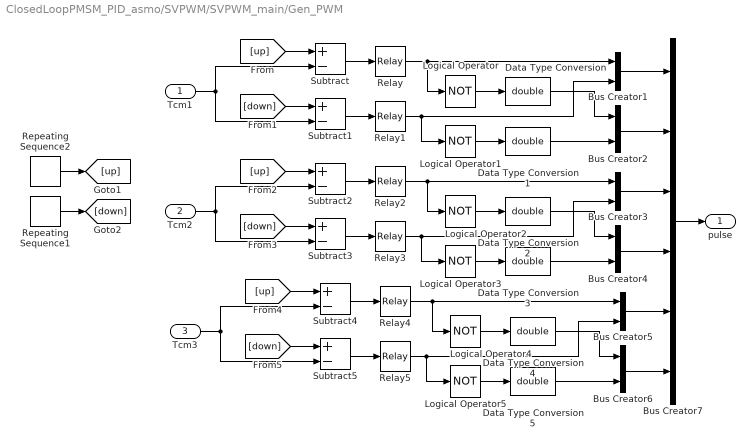
== system ClosedLoopPMSM_PID_asmo/SVPWM/SVPWM_main/Gen_PWM ==
  Tcm1 : Inport
  Tcm2 : Inport  Port=2
  Tcm3 : Inport  Port=3
  Bus Creator{1..6} (6 alike) : BusCreator  Inputs=2
  Bus Creator7 : BusCreator  Inputs=6
  Data Type Conversion{,1..5} (6 alike) : DataTypeConversion  OutDataTypeStr=double  SaturateOnIntegerOverflow=off  RndMeth=Floor
  Logical Operator{,1..5} (6 alike) : Logic  Operator=NOT  AllPortsSameDT=off
  Relay{,1..5} (6 alike) : Relay
  Repeating Sequence1 : simulink/Sources/Repeating Sequence  rep_seq_t=[0 Tpwm/2 Tpwm]  rep_seq_y=[Tpwm/4 Tpwm/2 Tpwm/4]
  Repeating Sequence2 : simulink/Sources/Repeating Sequence  rep_seq_t=[0 Tpwm/2 Tpwm]  rep_seq_y=[0 Tpwm/4 0]
  Subtract{,1..5} (6 alike) : Sum  Inputs=+-
  pulse : Outport
  wires:
  Relay1/1 -> Bus Creator1/2, Logical Operator1/1
  Relay/1 -> Bus Creator1/1, Logical Operator/1
  Logical Operator/1 -> Data Type Conversion/1
  Logical Operator1/1 -> Data Type Conversion1/1
  Subtract1/1 -> Relay1/1
  Subtract/1 -> Relay/1
  Bus Creator1/1 -> Bus Creator7/1
  Bus Creator2/1 -> Bus Creator7/2
  Bus Creator7/1 -> pulse/1
  Repeating Sequence2/1 -> [up]
  Tcm1/1 -> Subtract/2, Subtract1/2
  Repeating Sequence1/1 -> [down]
  [up] -> Subtract/1
  [down] -> Subtract1/1
  Data Type Conversion1/1 -> Bus Creator2/2
  Data Type Conversion/1 -> Bus Creator2/1
  Tcm2/1 -> Subtract2/2, Subtract3/2
  Subtract3/1 -> Relay3/1
  Bus Creator3/1 -> Bus Creator7/3
  Bus Creator4/1 -> Bus Creator7/4
  Relay2/1 -> Bus Creator3/1, Logical Operator2/1
  Logical Operator2/1 -> Data Type Conversion2/1
  Relay3/1 -> Bus Creator3/2, Logical Operator3/1
  [up] -> Subtract2/1
  Subtract2/1 -> Relay2/1
  [down] -> Subtract3/1
  Data Type Conversion2/1 -> Bus Creator4/1
  Tcm3/1 -> Subtract4/2, Subtract5/2
  Subtract5/1 -> Relay5/1
  Bus Creator5/1 -> Bus Creator7/5
  Bus Creator6/1 -> Bus Creator7/6
  Relay4/1 -> Bus Creator5/1, Logical Operator4/1
  Logical Operator4/1 -> Data Type Conversion4/1
  Relay5/1 -> Bus Creator5/2, Logical Operator5/1
  [up] -> Subtract4/1
  Subtract4/1 -> Relay4/1
  [down] -> Subtract5/1
  Data Type Conversion4/1 -> Bus Creator6/1
  Data Type Conversion3/1 -> Bus Creator4/2
  Data Type Conversion5/1 -> Bus Creator6/2
  Logical Operator5/1 -> Data Type Conversion5/1
  Logical Operator3/1 -> Data Type Conversion3/1

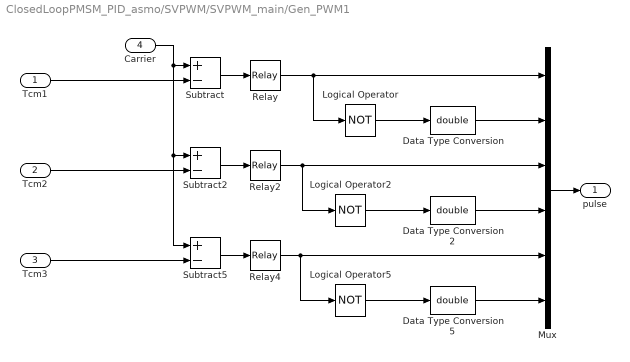
== system ClosedLoopPMSM_PID_asmo/SVPWM/SVPWM_main/Gen_PWM1 ==
  Tcm1 : Inport
  Tcm2 : Inport  Port=2
  Tcm3 : Inport  Port=3
  Carrier : Inport  Port=4
  Data Type Conversion : DataTypeConversion  OutDataTypeStr=double  SaturateOnIntegerOverflow=off  RndMeth=Floor
  Data Type Conversion2 : DataTypeConversion  OutDataTypeStr=double  SaturateOnIntegerOverflow=off  RndMeth=Floor
  Data Type Conversion5 : DataTypeConversion  OutDataTypeStr=double  SaturateOnIntegerOverflow=off  RndMeth=Floor
  Logical Operator : Logic  Operator=NOT  AllPortsSameDT=off
  Logical Operator2 : Logic  Operator=NOT  AllPortsSameDT=off
  Logical Operator5 : Logic  Operator=NOT  AllPortsSameDT=off
  Mux : Mux  Inputs=6
  Relay : Relay
  Relay2 : Relay
  Relay4 : Relay
  Subtract : Sum  Inputs=+-
  Subtract2 : Sum  Inputs=+-
  Subtract5 : Sum  Inputs=+-
  pulse : Outport
  wires:
  Relay/1 -> Mux/1, Logical Operator/1
  Logical Operator/1 -> Data Type Conversion/1
  Subtract/1 -> Relay/1
  Mux/1 -> pulse/1
  Tcm2/1 -> Subtract2/2
  Relay2/1 -> Logical Operator2/1, Mux/3
  Logical Operator2/1 -> Data Type Conversion2/1
  Tcm3/1 -> Subtract5/2
  Subtract5/1 -> Relay4/1
  Relay4/1 -> Logical Operator5/1, Mux/5
  Logical Operator5/1 -> Data Type Conversion5/1
  Tcm1/1 -> Subtract/2
  Carrier/1 -> Subtract5/1, Subtract2/1, Subtract/1
  Data Type Conversion5/1 -> Mux/6
  Data Type Conversion2/1 -> Mux/4
  Subtract2/1 -> Relay2/1
  Data Type Conversion/1 -> Mux/2

== matlab function ClosedLoopPMSM_PID_asmo/ASMO/back_emf_observer ==
  data: e_err_alpha input; de_est_alpha output; e_err_beta input; e_est_alpha input; e_est_beta input; we_hat input; de_est_beta output; dwe_hat output
function [de_est_alpha, de_est_beta, dwe_hat] = back_emf_observer( ...
    e_err_alpha, e_err_beta, e_est_alpha, e_est_beta, we_hat)

    % --- 1. THAM SO ---
    l_gain = 2e3;  % Tham so l quyet dinh toc do hoi tu 

    % --- 2. UOC LUONG TOC DO ---
    dwe_hat = (e_err_alpha * e_est_beta) - (e_err_beta * e_est_alpha);
    
    % --- 3. CAP NHAT BO QUAN SAT BACK-EMF ---
    % de_est_alpha/dt = -we_hat * e_est_beta - l * tilde_e_alpha 
    % de_est_beta/dt  =  we_hat * e_est_alpha - l * tilde_e_beta 
    
    de_est_alpha = (-we_hat * e_est_beta) - (l_gain * e_err_alpha); 
    de_est_beta  = ( we_hat * e_est_alpha) - (l_gain * e_err_beta);  
    
end

== matlab function ClosedLoopPMSM_PID_asmo/SVPWM/SVPWM_main/XYZ Calculate ==
  settings: fimath=|
      | fimath(...
      | 'RoundMode', 'floor',...
      | 'OverflowMode', 'wrap',...
      | 'ProductMode', 'KeepLSB', 'ProductWordLength', 32,...
      | 'SumMode', 'KeepLSB', 'SumWordLength', 32,...
      | 'CastBeforeSum', false)
  data: Ualpha input; XYZ output; Ubeta input; Udc input; Ts input
function XYZ = XYZ_calc(Ualpha, Ubeta, Udc, Ts)

k1 = sqrt(3) * Ubeta;
k2 = (sqrt(3)/2) * Ubeta;
k3 = 3/2 * Ualpha;

k = Ts / Udc;

X = k * (k1);
Y = k * (k2 + k3);
Z = k * (k2 - k3);

XYZ = [X, Y, Z];
end

== matlab function ClosedLoopPMSM_PID_asmo/ASMO/adaptive_gain ==
  data: k_alpha input; k_beta input; S_alpha input; S_beta input; H_alpha input; H_beta input; dk_alpha output; dk_beta output; dphi_alpha output; dphi_beta output; phi_alpha input; phi_beta input; K1_alpha input; K1_beta input; dK1_alpha output; dK1_beta output
function [dk_alpha, dk_beta, dphi_alpha, dphi_beta, dK1_alpha, dK1_beta] = adaptive_gain( ...
    k_alpha, k_beta, S_alpha, S_beta, H_alpha, H_beta, phi_alpha, phi_beta, K1_alpha, K1_beta)

    % Inputs:
    %   S_alpha, S_beta : Gia tri mat truot hien tai
    %   H_alpha, H_beta : Gia tri ham chuyen mach mem (tanh) hien tai
    %   k_alpha, k_beta : He so truot thich nghi k(t) cho buoc hien tai
    %   phi             : Gia tri hien tai cua phi 
    %   K1              : Gia tri luu tru cua K1 
    
    % Outputs:
    %   dk_apha, beta   : Dao ham theo thoi gian cua k_alpha, beta
    %   dphi            : Dao ham theo thoi gian cua phi (dphi/dt)
    %   dK1             : Dao ham cua bien nho K1
    
    %% Tham so
    K0      = 150;            % Toc do thich nghi
    tau     = 0.001;         % Hang so thoi gian bo loc
    epsilon = 0.5;            % Nguong xac dinh S gan 0
    gamma   = 1000;            % He so hoi tu nhanh ve gia tri K mong muon khi toi mat truot
    % GIOI HAN AN TOAN (Tranh k tang len vo cuc)
    MAX_K_DERIVATIVE = 100000; 
    MAX_K_VAL = 1500; % Neu k hien tai > 5000 thi ngung tang

    %% Tinh dao ham cua bo loc phi (Low-pass filter dynamics)
    % dphi/dt = (H - phi) / tau
    dphi_alpha = (H_alpha - phi_alpha) / tau;
    dphi_beta = (H_beta - phi_beta) / tau;

    %% Tinh dao ham cua he so k va K1 (Adaptive Law)
    if abs(S_alpha) > epsilon
        % --- Giai doan 1: Reaching Phase (|S| != 0) ---
        % dk/dt = K0 * |S|
        if k_alpha > MAX_K_VAL
            dk_alpha = 0; % Ngat tich phan neu k qua lon
        else
            dk_alpha = K0 * abs(S_alpha);
        end
        % Dat dK1/dt = dk/dt de K1 luon cap nhat bang k.
        dK1_alpha = dk_alpha;      
    else
        % --- Giai doan 2: Sliding Phase (|S| = 0) ---
        % k(t) = K1 * sqrt(|phi|)
        target_k_alpha = K1_alpha * sqrt(abs(phi_alpha));
        % dk/dt = gamma * (Target - Current)
        raw_dk_alpha = gamma * (target_k_alpha - k_alpha);
        % Bao hoa dao ham (tranh shock)
        dk_alpha = max(min(raw_dk_alpha, MAX_K_DERIVATIVE), -MAX_K_DERIVATIVE);
        % Trong giai doan nay, K1 giu nguyen gia tri
        dK1_alpha = 0;
    end

    if abs(S_beta) > epsilon
        % --- Giai doan 1: Reaching Phase (|S| != 0) ---
        % dk/dt = K0 * |S|
        if k_beta > MAX_K_VAL
            dk_beta = 0; 
        else
            dk_beta = K0 * abs(S_beta);
        end
        % Dat dK1/dt = dk/dt de K1 luon cap nhat bang k.      
        dK1_beta = dk_beta;
    else
        % --- Giai doan 2: Sliding Phase (|S| = 0) ---
        % k(t) = K1 * sqrt(|phi|)
        target_k_beta = K1_beta * sqrt(abs(phi_beta));
        % dk/dt = gamma * (Target - Current)
        raw_dk_beta = gamma * (target_k_beta - k_beta);
        % Bao hoa dao ham (tranh shock)
        dk_beta = max(min(raw_dk_beta, MAX_K_DERIVATIVE), -MAX_K_DERIVATIVE);
        % Trong giai doan nay, K1 giu nguyen gia tri
        dK1_beta = 0;
    end
end

== matlab function ClosedLoopPMSM_PID_asmo/SVPWM/SVPWM_main/T1T2 Calculate ==
  settings: fimath=|
      | fimath(...
      | 'RoundMode', 'floor',...
      | 'OverflowMode', 'wrap',...
      | 'ProductMode', 'KeepLSB', 'ProductWordLength', 32,...
      | 'SumMode', 'KeepLSB', 'SumWordLength', 32,...
      | 'CastBeforeSum', false)
  data: N input; T1 output; XYZ input; Tpwm input; T2 output
function [T1, T2] = T1T2_calc(N, XYZ, Tpwm)

    X = XYZ(1);
    Y = XYZ(2);
    Z = XYZ(3);

    % Default
    T1 = 0;
    T2 = 0;

    switch N
        case 1
            T1 = Z;   T2 = Y;
        case 2
            T1 = Y;   T2 = -X;
        case 3
            T1 = -Z;  T2 = X;
        case 4
            T1 = -X;  T2 = Z;
        case 5
            T1 = X;  T2 = -Y;
        case 6
            T1 = -Y;   T2 = -Z;
        otherwise
    end

    % Chuan hoa de dam bao T1 + T2 <= Tpwm
    if (T1 + T2) > Tpwm && (T1 + T2) > 0
        T1 = Tpwm * T1 / (T1 + T2);
        T2 = Tpwm * T2 / (T1 + T2);
    end
end

== matlab function ClosedLoopPMSM_PID_asmo/SVPWM/SVPWM_main/Tcm Calculate ==
  settings: fimath=|
      | fimath(...
      | 'RoundMode', 'floor',...
      | 'OverflowMode', 'wrap',...
      | 'ProductMode', 'KeepLSB', 'ProductWordLength', 32,...
      | 'SumMode', 'KeepLSB', 'SumWordLength', 32,...
      | 'CastBeforeSum', false)
  data: N input; Tcm1 output; T1 input; T2 input; Tcm2 output; Tpwm input; Tcm3 output
function [Tcm1, Tcm2, Tcm3] = Tcm_calc(N, T1, T2, Tpwm)
%Chuan hoa qua duty
a = (Tpwm - T1 - T2)/4; %T0/4
b = a + 0.5*T1;         %T0/4+T1/2
c = b + 0.5*T2;         %T0/4+T1/2+T2/2

% Gan theo sector
switch N
    case 1
        Tcm1 = b; Tcm2 = a; Tcm3 = c;
    case 2
        Tcm1 = a; Tcm2 = c; Tcm3 = b;
    case 3
        Tcm1 = a; Tcm2 = b; Tcm3 = c;
    case 4
        Tcm1 = c; Tcm2 = b; Tcm3 = a;
    case 5
        Tcm1 = c; Tcm2 = a; Tcm3 = b;
    case 6
        Tcm1 = b; Tcm2 = c; Tcm3 = a;
    otherwise
        Tcm1 = 0; Tcm2 = 0; Tcm3 = 0;
end

end

== matlab function ClosedLoopPMSM_PID_asmo/ASMO/current_observer ==
  data: S_alpha output; S_beta output; H_alpha output; H_beta output; e_err_alpha output; e_err_beta output; k_alpha input; k_beta input; di_est_alpha output; di_est_beta output; i_err_alpha output; i_err_beta output; ualpha input; ubeta input; ialpha input; ibeta input; Rs input; Ls input; e_est_alpha input; e_est_beta input; i_est_alpha input; i_est_beta input; int_e_alpha input; int_e_beta input
function [S_alpha, S_beta, H_alpha, H_beta, e_err_alpha, e_err_beta, di_est_alpha, di_est_beta, i_err_alpha, i_err_beta] = ...
    current_observer( k_alpha, k_beta, ualpha, ubeta, ialpha, ibeta, Rs, Ls, e_est_alpha, e_est_beta, i_est_alpha, i_est_beta, int_e_alpha, int_e_beta)

    % Inputs:
    %   ualpha, ubeta       : Dien ap do duoc (Stator voltage)
    %   ialpha, ibeta       : Dong dien do duoc (Measured current)
    %   Rs, Ls              : Dien tro va dien cam Stator
    %   i_est_alpha, beta   : Dong dien uoc luong (Estimated current) 
    %   int_e_alpha, beta   : Tich phan sai so dong dien (Integral of current error) 
    %   e_est_alpha, beta   : Back-EMF uoc luong (tu Back-EMF Observer 
    %   k_alpha, k_beta     : He so truot thich nghi (Adaptive gain) 
    
    % Outputs:
    %   di_est_alpha, beta  : Dao ham dong dien uoc luong 
    %   dk_alpha, beta      : Dao ham he so k 
    %   e_err_alpha, beta   : Sai so Back-EMF 
    %   S_alpha, S_beta     : Gia tri mat truot hien tai
    %   H_alpha, H_beta     : Gia tri ham chuyen mach mem (tanh) hien tai

    %% Tham so
    chi    = 15;    %giam rung, tang toc do hoi tu
    a      = 8;     %do day lop bien -> tang toc do hoi tu 

    %% Tinh toan sai so dong dien va back-EMF uoc luong
    % i_err = i_est - i_meas
    i_err_alpha = i_est_alpha - ialpha;
    i_err_beta  = i_est_beta  - ibeta;

    e_err_alpha = (chi*Ls - Rs) * i_err_alpha;
    e_err_beta = (chi*Ls - Rs) * i_err_beta;

    %% Tinh toan ham truot 
    % S = i_err + lambda * integral(i_err)
    S_alpha = i_err_alpha + chi * int_e_alpha;
    S_beta  = i_err_beta  + chi * int_e_beta;

    %% Ham chuyen mach 
    % H(S) = (e^(a*S) - e^(-a*S)) / (e^(a*S) + e^(-a*S))
    % H_alpha = (exp(a * S_alpha) - exp(-a * S_alpha)) / (exp(a * S_alpha) + exp(-a * S_alpha));
    % H_beta  = (exp(a * S_beta) - exp(-a * S_beta)) / (exp(a * S_beta) + exp(-a * S_beta));
    
    % H_alpha = tanh(a * S_alpha);
    % H_beta  = tanh(a * S_beta);
    % % H(S) = (2 / (1 + e^(-a*S))) - 1
    H_alpha = (2 / (1 + exp(-a * S_alpha))) - 1;
    H_beta  = (2 / (1 + exp(-a * S_beta))) - 1;

    %% Tinh toan dao ham dong dien uoc luong
    % di_est/dt = -Rs * i_est/Ls  + 1/Ls * (u - e_est) - k * H/Ls
    di_est_alpha = (-Rs * i_est_alpha/Ls ) + ualpha/Ls - e_est_alpha/Ls - k_alpha * H_alpha/Ls;
    di_est_beta  = (-Rs * i_est_beta/Ls )  + ubeta/Ls - e_est_beta/Ls - k_beta * H_beta/Ls;

end

== matlab function ClosedLoopPMSM_PID_asmo/SVPWM/SVPWM_main/Sector Calculate ==
  settings: fimath=|
      | fimath(...
      | 'RoundMode', 'floor',...
      | 'OverflowMode', 'wrap',...
      | 'ProductMode', 'KeepLSB', 'ProductWordLength', 32,...
      | 'SumMode', 'KeepLSB', 'SumWordLength', 32,...
      | 'CastBeforeSum', false)
  data: Valpha input; N output; Vbeta input
function N = sector_identification(Valpha, Vbeta)

    % DK A
    if Vbeta > 0
        A = 1;
    else
        A = 0;
    end

    % DK B
    if (sqrt(3)*Valpha - Vbeta) > 0
        B = 1;
    else
        B = 0;
    end

    %DK C
    if (-sqrt(3)*Valpha - Vbeta) > 0
        C = 1;
    else
        C = 0;
    end

    % Tinh sector
    N = A + 2*B + 4*C;
end
